simulink model "model3_bode_2021a"  (R2021a)
settings: Solver=VariableStepAuto  StartTime=0.0  StopTime=20  RelTol=1e-3
undefined symbols (not defined in the file or in its folder): car, disturb, E2TD, E2TN, T2VD
settings Model: Creator=Jirapu  LastModifiedBy=Jirapu
settings DebuggingCC: UnconnectedInputMsg=none  UnconnectedOutputMsg=none  UnconnectedLineMsg=none
settings RTWCC: DLArmComputeVersion=20.02.1

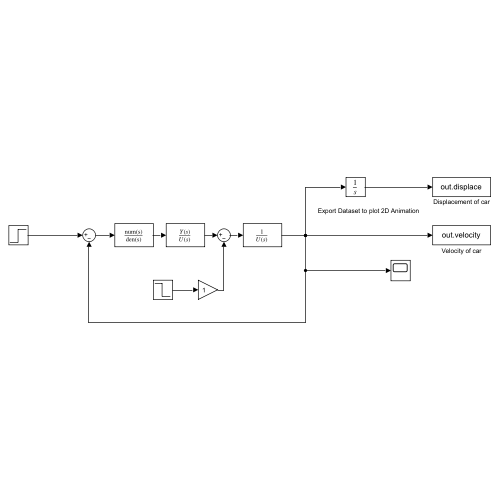
[thumbnail: Simulink's stored preview of the top-level diagram]
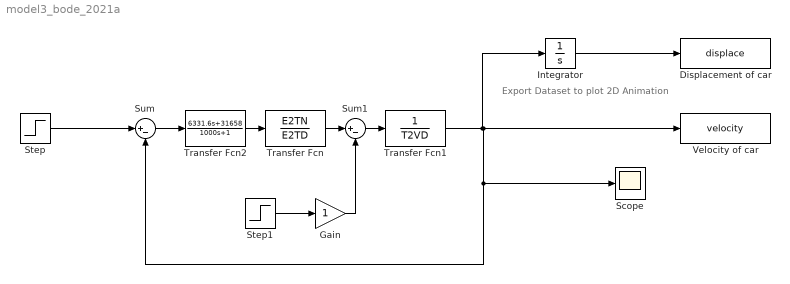
== system model3_bode_2021a ==
  note: Export Dataset to plot 2D Animation
  Displacement of car : ToWorkspace  VariableName=displace  SampleTime=0.03
  Gain : Gain
  Integrator : Integrator
  Scope : Scope
  Step : Step  Time=0  After=car.V_desire  SampleTime=0
  Step1 : Step  Time=0  After=disturb  SampleTime=0
  Sum : Sum  Inputs=|+-
  Sum1 : Sum  Inputs=|+-
  Transfer Fcn : TransferFcn  Numerator=E2TN  Denominator=E2TD
  Transfer Fcn1 : TransferFcn  Denominator=T2VD
  Transfer Fcn2 : TransferFcn  Numerator=[6331.6 31658]  Denominator=[1000 1]
  Velocity of car : ToWorkspace  VariableName=velocity  SampleTime=0.03
  wires:
  Transfer Fcn1/1 -> Velocity of car/1, Sum/2, Scope/1, Integrator/1
  Step1/1 -> Gain/1
  Transfer Fcn/1 -> Sum1/1
  Step/1 -> Sum/1
  Gain/1 -> Sum1/2
  Sum1/1 -> Transfer Fcn1/1
  Transfer Fcn2/1 -> Transfer Fcn/1
  Sum/1 -> Transfer Fcn2/1
  Integrator/1 -> Displacement of car/1
